simulink model "Aufgabe_9"  (Simulink 9.2)
settings: Solver=ode45  StartTime=0.0  StopTime=100.0  RelTol=1e-3  EnableMultiTasking=on
InitFcn:
  | t_save = 0.1
libraries: dspnetwork x9, simulink x2
settings Model: Creator=ST  LastModifiedBy=fleic
settings SolverCC: ZeroCrossAlgorithm=Adaptive
settings DataIOCC: SignalLoggingSaveFormat=Dataset
settings DebuggingCC: SolverPrmCheckMsg=warning  FcnCallInpInsideContextMsg=error
settings GRTTargetCC: CombineOutputUpdateFcns=on  GRTInterface=off
settings ConfigComp: CovSFcnEnable=off

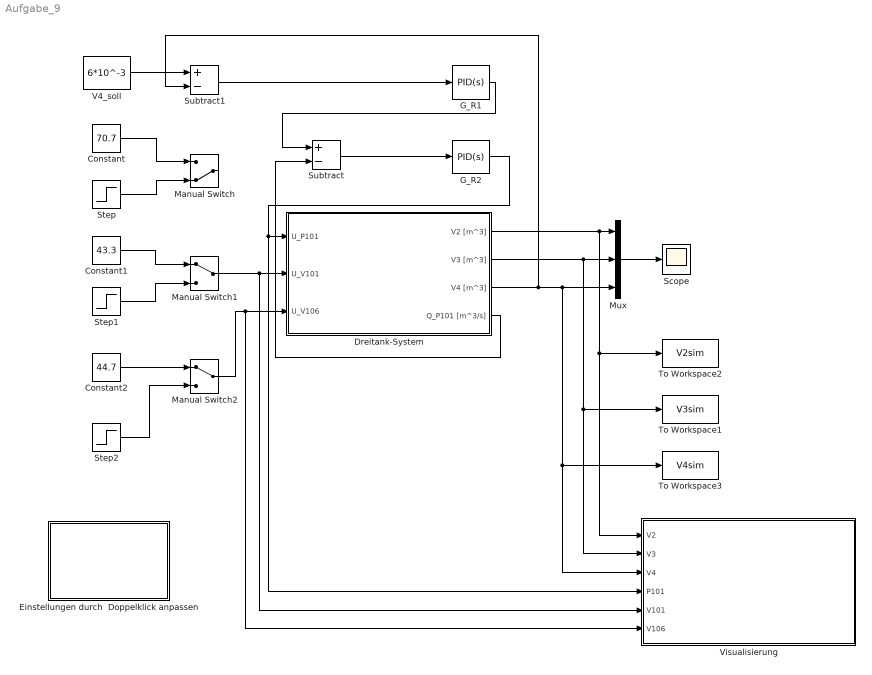
== system Aufgabe_9 ==
  Constant : Constant  Value=70.7
  Constant1 : Constant  Value=43.3
  Constant2 : Constant  Value=44.7
  Dreitank-System : Subsystem  mask{B101_Volumen=80*10^-3, B102_Initial_Volumen=8*10^-3, B103_Initial_Volumen=6*10^-3, B104_Initial_Volumen=5*10^-3, Querschnitt_Rohr_B102_B103=600*10^-6, Querschnitt_Rohr_B103_B104=600*10^-6, Flaeche_Behaelter=0.029}
      mask prompts: B101_Volumen "Volumen im Behälter B101 in m^3"; B102_Initial_Volumen "Initialvolumen im Behälter B102 in m^3"; B103_Initial_Volumen "Initialvolumen im Behälter B103 in m^3"; B104_Initial_Volumen "Initialvolumen im Behälter B104 in m^3"; Querschnitt_Rohr_B102_B103 "Rohrquerschnitt zwischen Behälter B102 und B103 in m^2"; Querschnitt_Rohr_B103_B104 "Rohrquerschnitt zwischen Behälter B103 und B104 in m^2"; Flaeche_Behaelter "Fläche der Behälter in m^2"
  Einstellungen durch  Doppelklick anpassen : MATLAB Function  InitFcn=tic  TreatAsAtomicUnit=on  mask{Auswahl=Bearbeiten}
      mask init:
      | maskStr = get_param(gcb,'Auswahl');
      | 
      | if strcmp(maskStr(1),'I')
      |      assignin('base','Testen',0)
      | else if strcmp(maskStr(1),'M')
      |         assignin('base','Testen',1)
      |     else
      |         assignin('base','Testen',2)
      |     end
      | end
  G_R1 : simulink/Continuous/PID Controller  Controller=PID  Form=Parallel  TimeDomain=Continuous-time  SampleTime=-1  IntegratorMethod=Forward Euler  FilterMethod=Forward Euler  ControllerParametersSource=internal  P=60  I=1  D=0  UseFilter=on  N=100  TunerSelectOption=Transfer Function Based (PID Tuner App)  InitialConditionSource=internal  InitialConditionForIntegrator=0  InitialConditionForFilter=0  DifferentiatorICPrevScaledInput=0  ExternalReset=none  TrackingMode=off  Kt=1  LimitOutput=off  UpperSaturationLimit=inf  LowerSaturationLimit=-inf  LinearizeAsGain=on  AntiWindupMode=none  Kb=1  POutMin=[]  POutMax=[]  IOutMin=[]  IOutMax=[]  DOutMin=[]  DOutMax=[]  NOutMin=[]  NOutMax=[]  SumOutMin=[]  SumOutMax=[]  SaturationOutMin=[]  SaturationOutMax=[]  PParamMin=[]  PParamMax=[]  IParamMin=[]  IParamMax=[]  DParamMin=[]  DParamMax=[]  NParamMin=[]  NParamMax=[]  KbParamMin=[]  KbParamMax=[]  KtParamMin=[]  KtParamMax=[]  KbOutMin=[]  KbOutMax=[]  KtOutMin=[]  KtOutMax=[]  IntegratorOutMin=[]  IntegratorOutMax=[]  FilterOutMin=[]  FilterOutMax=[]  SumI1OutMin=[]  SumI1OutMax=[]  SumI2OutMin=[]  SumI2OutMax=[]  SumI3OutMin=[]  SumI3OutMax=[]  SumI4OutMin=[]  SumI4OutMax=[]  SumDOutMin=[]  SumDOutMax=[]  DifferentiatorOutMin=[]  DifferentiatorOutMax=[]  FilterDiffOutCoefMin=[]  FilterDiffOutCoefMax=[]  ReciprocalOutMin=[]  ReciprocalOutMax=[]  SumDenOutMin=[]  SumDenOutMax=[]  SumNumOutMin=[]  SumNumOutMax=[]  DivideOutMin=[]  DivideOutMax=[]  IntegratorContinuousStateAttributes=''  IntegratorStateMustResolveToSignalObject=off  IntegratorRTWStateStorageClass=Auto  FilterContinuousStateAttributes=''  FilterStateMustResolveToSignalObject=off  FilterRTWStateStorageClass=Auto  ParallelPVariant=InternalParameters  IdealPVariant=Disabled  IVariant=InternalParameters  DVariant=InternalParameters  IntegratorVariant=Continuous  SatVariant=Disabled  AWVariant=Passthrough  PCopyVariant=Disabled  TRVariant=Disabled  FdbkBlocksVariant=Forward  IdealPFdbkVariant=Disabled  SatFdbkVariant=Disabled  DerivativeFilterVariant=ContFilter  NVariant=InternalParameters  NCopyVariant=Disabled  FilterICVariant=InternalICsFilter  IntegratorICVariant=InternalICs  ExternalResetVariant=Disabled  TRSumVariant=Passthrough  SumFdbkVariant=Disabled  SumVariant=Sum_PID
  "G_R2 " : simulink/Continuous/PID Controller  Controller=PID  Form=Parallel  TimeDomain=Continuous-time  SampleTime=-1  IntegratorMethod=Forward Euler  FilterMethod=Forward Euler  ControllerParametersSource=internal  P=469*50  I=469  D=0  UseFilter=on  N=100  TunerSelectOption=Transfer Function Based (PID Tuner App)  InitialConditionSource=internal  InitialConditionForIntegrator=0  InitialConditionForFilter=0  DifferentiatorICPrevScaledInput=0  ExternalReset=none  TrackingMode=off  Kt=1  LimitOutput=off  UpperSaturationLimit=inf  LowerSaturationLimit=-inf  LinearizeAsGain=on  AntiWindupMode=none  Kb=1  POutMin=[]  POutMax=[]  IOutMin=[]  IOutMax=[]  DOutMin=[]  DOutMax=[]  NOutMin=[]  NOutMax=[]  SumOutMin=[]  SumOutMax=[]  SaturationOutMin=[]  SaturationOutMax=[]  PParamMin=[]  PParamMax=[]  IParamMin=[]  IParamMax=[]  DParamMin=[]  DParamMax=[]  NParamMin=[]  NParamMax=[]  KbParamMin=[]  KbParamMax=[]  KtParamMin=[]  KtParamMax=[]  KbOutMin=[]  KbOutMax=[]  KtOutMin=[]  KtOutMax=[]  IntegratorOutMin=[]  IntegratorOutMax=[]  FilterOutMin=[]  FilterOutMax=[]  SumI1OutMin=[]  SumI1OutMax=[]  SumI2OutMin=[]  SumI2OutMax=[]  SumI3OutMin=[]  SumI3OutMax=[]  SumI4OutMin=[]  SumI4OutMax=[]  SumDOutMin=[]  SumDOutMax=[]  DifferentiatorOutMin=[]  DifferentiatorOutMax=[]  FilterDiffOutCoefMin=[]  FilterDiffOutCoefMax=[]  ReciprocalOutMin=[]  ReciprocalOutMax=[]  SumDenOutMin=[]  SumDenOutMax=[]  SumNumOutMin=[]  SumNumOutMax=[]  DivideOutMin=[]  DivideOutMax=[]  IntegratorContinuousStateAttributes=''  IntegratorStateMustResolveToSignalObject=off  IntegratorRTWStateStorageClass=Auto  FilterContinuousStateAttributes=''  FilterStateMustResolveToSignalObject=off  FilterRTWStateStorageClass=Auto  ParallelPVariant=InternalParameters  IdealPVariant=Disabled  IVariant=InternalParameters  DVariant=InternalParameters  IntegratorVariant=Continuous  SatVariant=Disabled  AWVariant=Passthrough  PCopyVariant=Disabled  TRVariant=Disabled  FdbkBlocksVariant=Forward  IdealPFdbkVariant=Disabled  SatFdbkVariant=Disabled  DerivativeFilterVariant=ContFilter  NVariant=InternalParameters  NCopyVariant=Disabled  FilterICVariant=InternalICsFilter  IntegratorICVariant=InternalICs  ExternalResetVariant=Disabled  TRSumVariant=Passthrough  SumFdbkVariant=Disabled  SumVariant=Sum_PID
  Manual Switch : ManualSwitch  CurrentSetting=0
  Manual Switch1 : ManualSwitch
  Manual Switch2 : ManualSwitch
  Mux : Mux  Inputs=3
  Scope : Scope
  Step : Step  Before=70.7  After=80.7  SampleTime=0
  Step1 : Step  Before=43.3  After=53.3  SampleTime=0
  Step2 : Step  Before=44.7  After=54.7  SampleTime=0
  Subtract : Sum  Inputs=+-
  Subtract1 : Sum  Inputs=+-
  To Workspace1 : ToWorkspace  VariableName=V3sim  SampleTime=t_save
  To Workspace2 : ToWorkspace  VariableName=V2sim  SampleTime=t_save
  To Workspace3 : ToWorkspace  VariableName=V4sim  SampleTime=t_save
  "V4_soll " : Constant  Value=6*10^-3
  Visualisierung : Subsystem
      settings: OpenFcn=|
      | !Dreitank_Visualisierung_64bit\Dreitank.blend.exe
      | !Dreitank_Visualisierung_32bit\Dreitank.blend.exe
  wires:
  Dreitank-System/1(V2 [m^3]) -> Visualisierung/1(V2), To Workspace2/1, Mux/1
  Dreitank-System/2(V3 [m^3]) -> Visualisierung/2(V3), To Workspace1/1, Mux/2
  Dreitank-System/3(V4 [m^3]) -> Subtract1/2, Visualisierung/3(V4), To Workspace3/1, Mux/3
  Mux/1 -> Scope/1
  Constant/1 -> Manual Switch/1
  Step/1 -> Manual Switch/2
  Manual Switch1/1 -> Dreitank-System/2("U_V101 "), Visualisierung/5(V101)
  Constant1/1 -> Manual Switch1/1
  Step1/1 -> Manual Switch1/2
  Constant2/1 -> Manual Switch2/1
  Step2/1 -> Manual Switch2/2
  Manual Switch2/1 -> Visualisierung/6(V106), Dreitank-System/3(U_V106)
  Dreitank-System/4(Q_P101 [m^3/s]) -> Subtract/2
  Subtract/1 -> "G_R2 "/1
  "G_R2 "/1 -> Visualisierung/4(P101), Dreitank-System/1(U_P101)
  "V4_soll "/1 -> Subtract1/1
  Subtract1/1 -> G_R1/1
  G_R1/1 -> Subtract/1

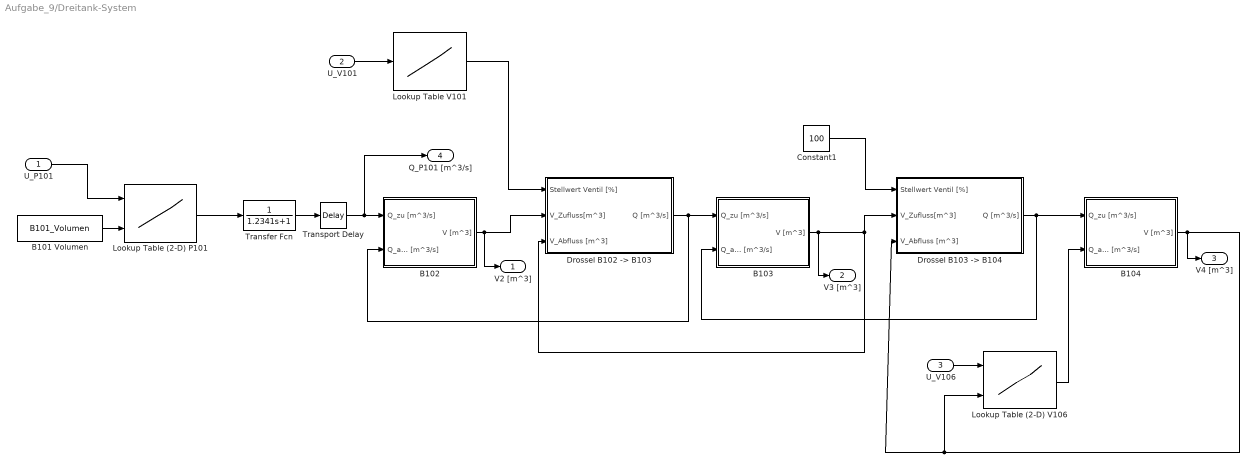
== system Aufgabe_9/Dreitank-System ==
  U_P101 : Inport
  "U_V101 " : Inport  Port=2
  U_V106 : Inport  Port=3
  B101 Volumen : Constant  Value=B101_Volumen  OutDataTypeStr=double
  B102 : Subsystem  mask{Initial_Volumen=B102_Initial_Volumen}
      mask prompts: Initial_Volumen "Initialvolumen"
  B103 : Subsystem  mask{Initial_Volumen=B103_Initial_Volumen}
      mask prompts: Initial_Volumen "Initialvolumen"
  B104 : Subsystem  mask{Initial_Volumen=B104_Initial_Volumen}
      mask prompts: Initial_Volumen "Initialvolumen"
  Constant1 : Constant  Value=100
  "Drossel B102 -> B103" : Subsystem  mask{Querschnitt_Rohr=Querschnitt_Rohr_B102_B103, Flaeche_Behaelter=Flaeche_Behaelter}
      mask prompts: Querschnitt_Rohr "Querschnitt des Rohrs in m^2"; Flaeche_Behaelter "Flaeche_Behaelter in m^2"
  "Drossel B103 -> B104" : Subsystem  mask{Querschnitt_Rohr=Querschnitt_Rohr_B102_B103, Flaeche_Behaelter=Flaeche_Behaelter}
      mask prompts: Querschnitt_Rohr "Querschnitt des Rohrs in m^2"; Flaeche_Behaelter "Flaeche_Behaelter in m^2"
  Lookup Table (2-D) P101 : Lookup2D  RowIndex=[50,55,60,65,70,75,80,85,90,95,100]  ColumnIndex=[40,130]*10^-3  Table=reshape([0,0.0606,0.2450,0.3378,0.4184,0.5002,0.5801,0.6551,0.7138,0.7746,0.8206,0,0.2799,0.3497,0.4278,0.5053,0.5810,0.6481,0.7168,0.7695,0.8350,0.8786]*10^-3,11,2)  LookUpMeth=Interpolation-Use End Values
  Lookup Table (2-D) V106 : Lookup2D  RowIndex=[15,20,25,30,35,40,45,50,55,60,65,70,75,80,85]  ColumnIndex=[2,2.8,10]*10^-3  Table=reshape([0,0,0,0,0,0,0,0,0,0,0,0,0,0,0,0,0.032,0.097,0.179,0.262,0.361,0.475,0.604,0.902,1.089,1.318,1.536,1.685,1.853,2.029,0,0.032,0.097,0.179,0.262,0.361,0.475,0.604,0.902,1.089,1.318,1.536,1.685,1.853,2.029]*10^-3,15,3)  LookUpMeth=Interpolation-Use End Values
  Lookup Table V101 : Lookup  InputValues=[0,20,25,30,35,40,45,50,55,60,65,70,75,80,85,90,100]  Table=[100,96,90,88,84,76,68,60,49,41,34,27,22,19,16,12,0]  LookUpMeth=Interpolation-Use End Values
  Transfer Fcn : TransferFcn  Denominator=[1.2341 1]
  Transport Delay : TransportDelay  DelayTime=1.1
  V2 [m^3] : Outport
  V3 [m^3] : Outport  Port=2
  V4 [m^3] : Outport  Port=3
  Q_P101 [m^3/s] : Outport  Port=4
  wires:
  "Drossel B103 -> B104"/1(Q [m^3/s]) -> B104/1(Q_zu [m^3/s]), B103/2(Q_ab [m^3/s])
  "Drossel B102 -> B103"/1(Q [m^3/s]) -> B102/2(Q_ab [m^3/s]), B103/1(Q_zu [m^3/s])
  B101 Volumen/1 -> Lookup Table (2-D) P101/2
  B103/1(V [m^3]) -> "Drossel B103 -> B104"/2(V_Zufluss[m^3]), "Drossel B102 -> B103"/3(V_Abfluss [m^3]), V3 [m^3]/1
  U_P101/1 -> Lookup Table (2-D) P101/1
  U_V106/1 -> Lookup Table (2-D) V106/1
  Lookup Table V101/1 -> "Drossel B102 -> B103"/1(Stellwert Ventil [%])
  Lookup Table (2-D) V106/1 -> B104/2(Q_ab [m^3/s])
  B102/1(V [m^3]) -> V2 [m^3]/1, "Drossel B102 -> B103"/2(V_Zufluss[m^3])
  "U_V101 "/1 -> Lookup Table V101/1
  B104/1(V [m^3]) -> Lookup Table (2-D) V106/2, "Drossel B103 -> B104"/3(V_Abfluss [m^3]), V4 [m^3]/1
  Constant1/1 -> "Drossel B103 -> B104"/1(Stellwert Ventil [%])
  Transfer Fcn/1 -> Transport Delay/1
  Lookup Table (2-D) P101/1 -> Transfer Fcn/1
  Transport Delay/1 -> Q_P101 [m^3/s]/1, B102/1(Q_zu [m^3/s])

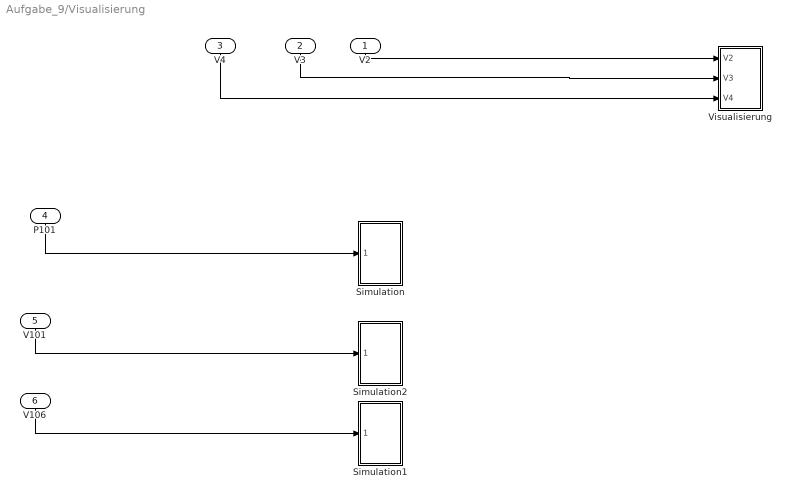
== system Aufgabe_9/Visualisierung ==
  V2 : Inport
  V3 : Inport  Port=2
  V4 : Inport  Port=3
  P101 : Inport  Port=4
  V101 : Inport  Port=5
  V106 : Inport  Port=6
  Simulation : Subsystem
  Simulation1 : Subsystem
  Simulation2 : Subsystem
  "Visualisierung " : Subsystem
      settings: OpenFcn=Visualisierung/Dreitank.exe
  wires:
  V106/1 -> Simulation1/1(ValveOne Value)
  V101/1 -> Simulation2/1(ValveTwo Value)
  V2/1 -> "Visualisierung "/1(V2)
  V4/1 -> "Visualisierung "/3("V4 ")
  P101/1 -> Simulation/1(PumpValue)
  V3/1 -> "Visualisierung "/2(V3)

== system Aufgabe_9/Dreitank-System/B102 ==
  Q_zu [m^3/s] : Inport
  Q_ab [m^3/s] : Inport  Port=2
  Integrator1 : Integrator  InitialCondition=Initial_Volumen  LimitOutput=on  UpperSaturationLimit=10*10^-3  LowerSaturationLimit=0  ContinuousStateAttributes='Volumen_B102'
  Sum : Sum  Inputs=|+-
  V [m^3] : Outport
  wires:
  Q_ab [m^3/s]/1 -> Sum/2
  Q_zu [m^3/s]/1 -> Sum/1
  Integrator1/1 -> V [m^3]/1
  Sum/1 -> Integrator1/1

== system Aufgabe_9/Dreitank-System/B103 ==
  Q_zu [m^3/s] : Inport
  Q_ab [m^3/s] : Inport  Port=2
  Integrator1 : Integrator  InitialCondition=Initial_Volumen  LimitOutput=on  UpperSaturationLimit=10*10^-3  LowerSaturationLimit=0  ContinuousStateAttributes='Volumen_B102'
  Sum : Sum  Inputs=|+-
  V [m^3] : Outport
  wires:
  Q_ab [m^3/s]/1 -> Sum/2
  Q_zu [m^3/s]/1 -> Sum/1
  Integrator1/1 -> V [m^3]/1
  Sum/1 -> Integrator1/1

== system Aufgabe_9/Dreitank-System/B104 ==
  Q_zu [m^3/s] : Inport
  Q_ab [m^3/s] : Inport  Port=2
  Integrator1 : Integrator  InitialCondition=Initial_Volumen  LimitOutput=on  UpperSaturationLimit=10*10^-3  LowerSaturationLimit=0  ContinuousStateAttributes='Volumen_B102'
  Sum : Sum  Inputs=|+-
  V [m^3] : Outport
  wires:
  Sum/1 -> Integrator1/1
  Integrator1/1 -> V [m^3]/1
  Q_zu [m^3/s]/1 -> Sum/1
  Q_ab [m^3/s]/1 -> Sum/2

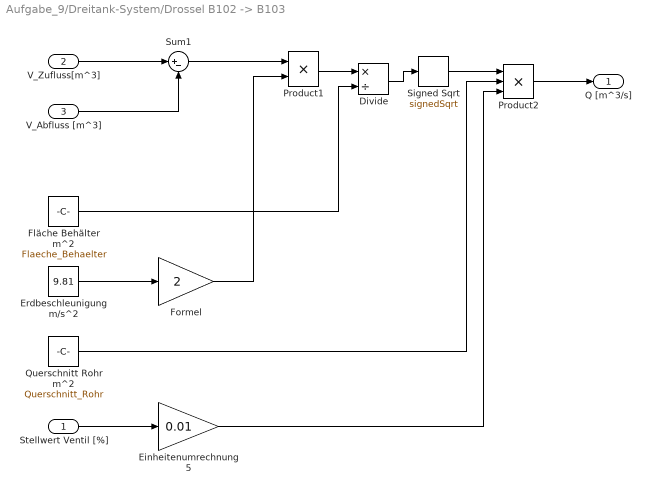
== system Aufgabe_9/Dreitank-System/Drossel B102 -> B103 ==
  Stellwert Ventil [%] : Inport
  V_Zufluss[m^3] : Inport  Port=2
  V_Abfluss [m^3] : Inport  Port=3
  Divide : Product  Inputs=*/
  Einheitenumrechnung 5 : Gain  Gain=0.01
  Erdbeschleunigung m/s^2 : Constant  Value=9.81  OutDataTypeStr=double
  Fläche Behälter m^2 : Constant  Value=Flaeche_Behaelter  OutDataTypeStr=double
  Formel : Gain  Gain=2
  Product1 : Product  RndMeth=Zero
  Product2 : Product  Inputs=3  RndMeth=Zero
  Querschnitt Rohr m^2 : Constant  Value=Querschnitt_Rohr  OutDataTypeStr=double
  Signed Sqrt : Sqrt  Operator=signedSqrt  SaturateOnIntegerOverflow=on
  Sum1 : Sum  Inputs=|+-
  Q [m^3/s] : Outport
  wires:
  Fläche Behälter m^2/1 -> Divide/2
  Divide/1 -> Signed Sqrt/1
  Product1/1 -> Divide/1
  Formel/1 -> Product1/2
  Sum1/1 -> Product1/1
  V_Abfluss [m^3]/1 -> Sum1/2
  V_Zufluss[m^3]/1 -> Sum1/1
  Product2/1 -> Q [m^3/s]/1
  Einheitenumrechnung 5/1 -> Product2/3
  Stellwert Ventil [%]/1 -> Einheitenumrechnung 5/1
  Querschnitt Rohr m^2/1 -> Product2/2
  Signed Sqrt/1 -> Product2/1
  Erdbeschleunigung m/s^2/1 -> Formel/1

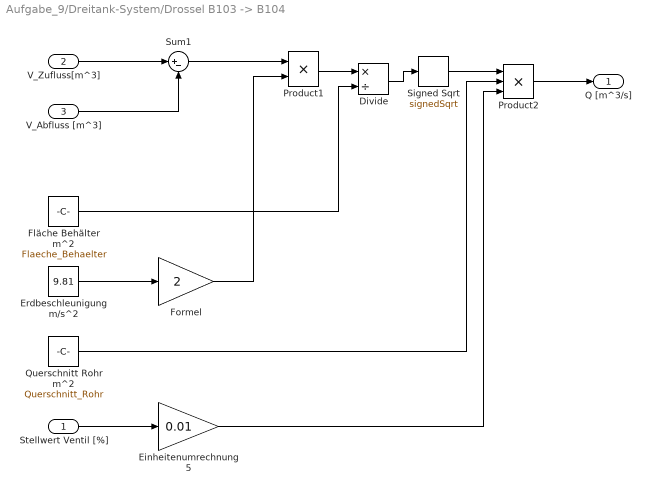
== system Aufgabe_9/Dreitank-System/Drossel B103 -> B104 ==
  Stellwert Ventil [%] : Inport
  V_Zufluss[m^3] : Inport  Port=2
  V_Abfluss [m^3] : Inport  Port=3
  Divide : Product  Inputs=*/
  Einheitenumrechnung 5 : Gain  Gain=0.01
  Erdbeschleunigung m/s^2 : Constant  Value=9.81  OutDataTypeStr=double
  Fläche Behälter m^2 : Constant  Value=Flaeche_Behaelter  OutDataTypeStr=double
  Formel : Gain  Gain=2
  Product1 : Product  RndMeth=Zero
  Product2 : Product  Inputs=3  RndMeth=Zero
  Querschnitt Rohr m^2 : Constant  Value=Querschnitt_Rohr  OutDataTypeStr=double
  Signed Sqrt : Sqrt  Operator=signedSqrt  SaturateOnIntegerOverflow=on
  Sum1 : Sum  Inputs=|+-
  Q [m^3/s] : Outport
  wires:
  Erdbeschleunigung m/s^2/1 -> Formel/1
  Signed Sqrt/1 -> Product2/1
  Querschnitt Rohr m^2/1 -> Product2/2
  Stellwert Ventil [%]/1 -> Einheitenumrechnung 5/1
  Einheitenumrechnung 5/1 -> Product2/3
  Product2/1 -> Q [m^3/s]/1
  V_Zufluss[m^3]/1 -> Sum1/1
  V_Abfluss [m^3]/1 -> Sum1/2
  Sum1/1 -> Product1/1
  Formel/1 -> Product1/2
  Product1/1 -> Divide/1
  Divide/1 -> Signed Sqrt/1
  Fläche Behälter m^2/1 -> Divide/2

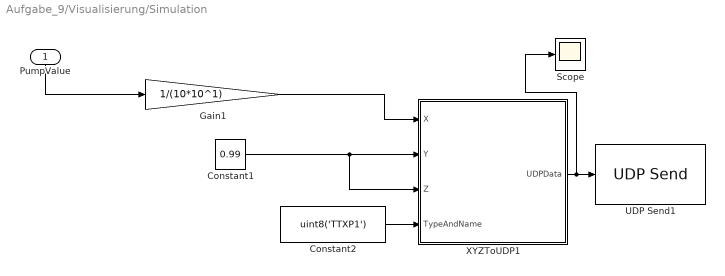
== system Aufgabe_9/Visualisierung/Simulation ==
  PumpValue : Inport
  Constant1 : Constant  Value=0.99
  Constant2 : Constant  Value=uint8('TTXP1')
  Gain1 : Gain  Gain=1/(10*10^1)
  Scope : Scope
  UDP Send1 : dspnetwork/UDP Send  remoteURL='localhost'  remotePort=9999  localURL='0.0.0.0'  localPortSource=Automatically determine  localPort=-1  sampletime=-1  blockPlatform=WINDOWS  separateLengthPort=0
      settings: SourceProductName=DSP System Toolbox  SourceProductBaseCode=DS
  XYZToUDP1 : Subsystem
  wires:
  XYZToUDP1/1(UDPData) -> Scope/1, UDP Send1/1
  Constant1/1 -> XYZToUDP1/3(Z), XYZToUDP1/2(Y)
  Constant2/1 -> XYZToUDP1/4(TypeAndName)
  PumpValue/1 -> Gain1/1
  Gain1/1 -> XYZToUDP1/1(X)

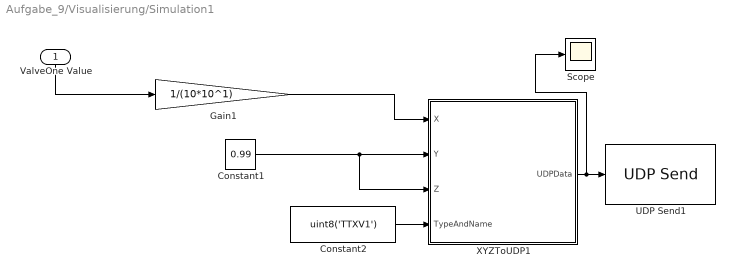
== system Aufgabe_9/Visualisierung/Simulation1 ==
  ValveOne Value : Inport
  Constant1 : Constant  Value=0.99
  Constant2 : Constant  Value=uint8('TTXV1')
  Gain1 : Gain  Gain=1/(10*10^1)
  Scope : Scope
  UDP Send1 : dspnetwork/UDP Send  remoteURL='localhost'  remotePort=9999  localURL='0.0.0.0'  localPortSource=Automatically determine  localPort=-1  sampletime=-1  blockPlatform=WINDOWS  separateLengthPort=0
      settings: SourceProductName=DSP System Toolbox  SourceProductBaseCode=DS
  XYZToUDP1 : Subsystem
  wires:
  XYZToUDP1/1(UDPData) -> Scope/1, UDP Send1/1
  Constant1/1 -> XYZToUDP1/3(Z), XYZToUDP1/2(Y)
  Constant2/1 -> XYZToUDP1/4(TypeAndName)
  ValveOne Value/1 -> Gain1/1
  Gain1/1 -> XYZToUDP1/1(X)

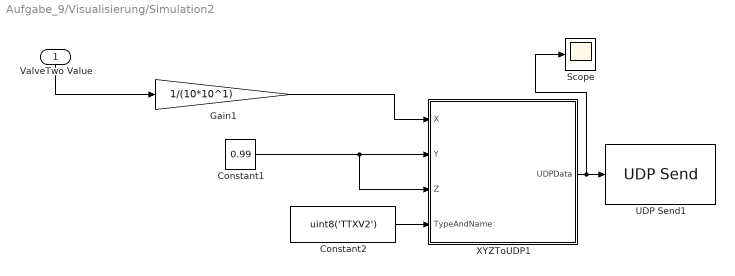
== system Aufgabe_9/Visualisierung/Simulation2 ==
  ValveTwo Value : Inport
  Constant1 : Constant  Value=0.99
  Constant2 : Constant  Value=uint8('TTXV2')
  Gain1 : Gain  Gain=1/(10*10^1)
  Scope : Scope
  UDP Send1 : dspnetwork/UDP Send  remoteURL='localhost'  remotePort=9999  localURL='0.0.0.0'  localPortSource=Automatically determine  localPort=-1  sampletime=-1  blockPlatform=WINDOWS  separateLengthPort=0
      settings: SourceProductName=DSP System Toolbox  SourceProductBaseCode=DS
  XYZToUDP1 : Subsystem
  wires:
  XYZToUDP1/1(UDPData) -> Scope/1, UDP Send1/1
  Constant1/1 -> XYZToUDP1/3(Z), XYZToUDP1/2(Y)
  Constant2/1 -> XYZToUDP1/4(TypeAndName)
  ValveTwo Value/1 -> Gain1/1
  Gain1/1 -> XYZToUDP1/1(X)

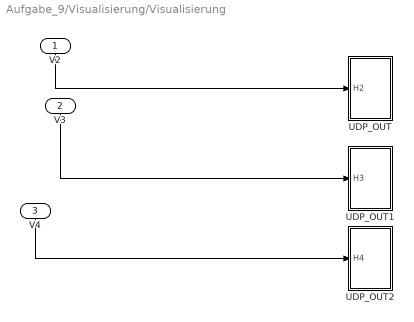
== system Aufgabe_9/Visualisierung/Visualisierung  ==
  V2 : Inport
  V3 : Inport  Port=2
  "V4 " : Inport  Port=3
  UDP_OUT : Subsystem
  UDP_OUT1 : Subsystem
  UDP_OUT2 : Subsystem
  wires:
  V2/1 -> UDP_OUT/1(H2)
  V3/1 -> UDP_OUT1/1(H3)
  "V4 "/1 -> UDP_OUT2/1(H4)

== system Aufgabe_9/Visualisierung/Simulation/XYZToUDP1 ==
  X : Inport
  Y : Inport  Port=2
  Z : Inport  Port=3
  TypeAndName : Inport  Port=4
  PrepareUDP_XYZ : MATLAB Function  TreatAsAtomicUnit=on
  UDPData : Outport
  wires:
  PrepareUDP_XYZ/1(UDPData) -> UDPData/1
  X/1 -> PrepareUDP_XYZ/1(DataX)
  TypeAndName/1 -> PrepareUDP_XYZ/4(TnName)
  Z/1 -> PrepareUDP_XYZ/3(DataZ)
  Y/1 -> PrepareUDP_XYZ/2(DataY)

== system Aufgabe_9/Visualisierung/Simulation1/XYZToUDP1 ==
  X : Inport
  Y : Inport  Port=2
  Z : Inport  Port=3
  TypeAndName : Inport  Port=4
  PrepareUDP_XYZ : MATLAB Function  TreatAsAtomicUnit=on
  UDPData : Outport
  wires:
  PrepareUDP_XYZ/1(UDPData) -> UDPData/1
  X/1 -> PrepareUDP_XYZ/1(DataX)
  TypeAndName/1 -> PrepareUDP_XYZ/4(TnName)
  Z/1 -> PrepareUDP_XYZ/3(DataZ)
  Y/1 -> PrepareUDP_XYZ/2(DataY)

== system Aufgabe_9/Visualisierung/Simulation2/XYZToUDP1 ==
  X : Inport
  Y : Inport  Port=2
  Z : Inport  Port=3
  TypeAndName : Inport  Port=4
  PrepareUDP_XYZ : MATLAB Function  TreatAsAtomicUnit=on
  UDPData : Outport
  wires:
  PrepareUDP_XYZ/1(UDPData) -> UDPData/1
  X/1 -> PrepareUDP_XYZ/1(DataX)
  TypeAndName/1 -> PrepareUDP_XYZ/4(TnName)
  Z/1 -> PrepareUDP_XYZ/3(DataZ)
  Y/1 -> PrepareUDP_XYZ/2(DataY)

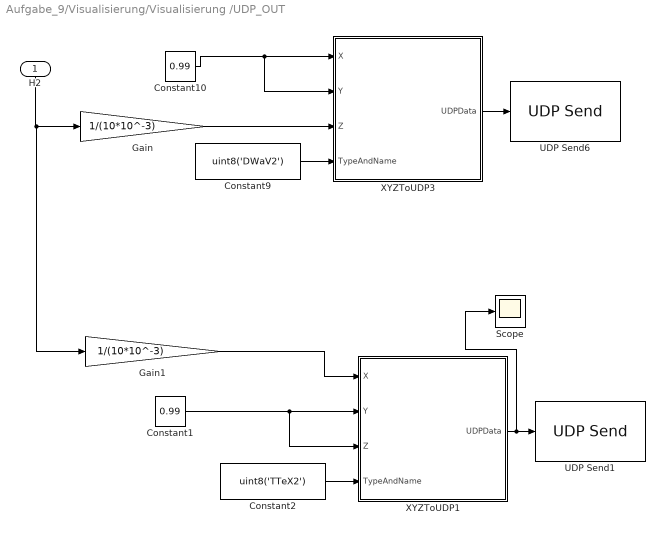
== system Aufgabe_9/Visualisierung/Visualisierung /UDP_OUT ==
  H2 : Inport
  Constant1 : Constant  Value=0.99
  Constant10 : Constant  Value=0.99
  Constant2 : Constant  Value=uint8('TTeX2')
  Constant9 : Constant  Value=uint8('DWaV2')
  Gain : Gain  Gain=1/(10*10^-3)
  Gain1 : Gain  Gain=1/(10*10^-3)
  Scope : Scope
  UDP Send1 : dspnetwork/UDP Send  remoteURL='localhost'  remotePort=9999  localURL='0.0.0.0'  localPortSource=Automatically determine  localPort=-1  sampletime=-1  blockPlatform=WINDOWS  separateLengthPort=0
      settings: SourceProductName=DSP System Toolbox  SourceProductBaseCode=DS
  UDP Send6 : dspnetwork/UDP Send  remoteURL='localhost'  remotePort=9999  localURL='0.0.0.0'  localPortSource=Automatically determine  localPort=-1  sampletime=-1  blockPlatform=WINDOWS  separateLengthPort=0
      settings: SourceProductName=DSP System Toolbox  SourceProductBaseCode=DS
  XYZToUDP1 : Subsystem
  XYZToUDP3 : Subsystem
  wires:
  XYZToUDP3/1(UDPData) -> UDP Send6/1
  Constant10/1 -> XYZToUDP3/1(X), XYZToUDP3/2(Y)
  Constant9/1 -> XYZToUDP3/4(TypeAndName)
  Gain/1 -> XYZToUDP3/3(Z)
  XYZToUDP1/1(UDPData) -> Scope/1, UDP Send1/1
  Constant1/1 -> XYZToUDP1/3(Z), XYZToUDP1/2(Y)
  Constant2/1 -> XYZToUDP1/4(TypeAndName)
  H2/1 -> Gain1/1, Gain/1
  Gain1/1 -> XYZToUDP1/1(X)

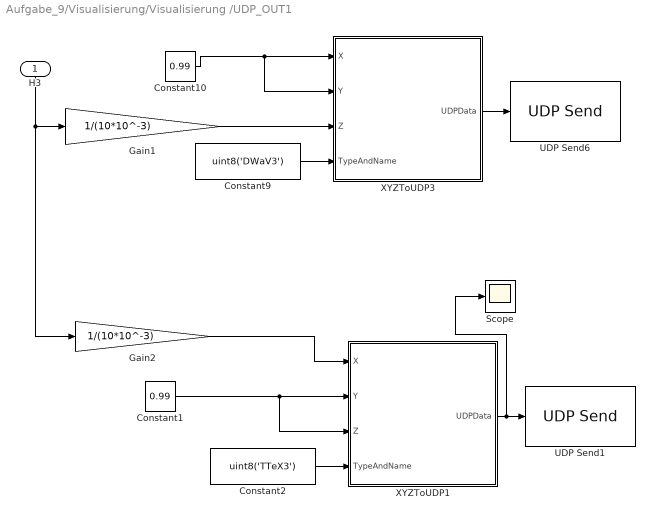
== system Aufgabe_9/Visualisierung/Visualisierung /UDP_OUT1 ==
  H3 : Inport
  Constant1 : Constant  Value=0.99
  Constant10 : Constant  Value=0.99
  Constant2 : Constant  Value=uint8('TTeX3')
  Constant9 : Constant  Value=uint8('DWaV3')
  Gain1 : Gain  Gain=1/(10*10^-3)
  Gain2 : Gain  Gain=1/(10*10^-3)
  Scope : Scope
  UDP Send1 : dspnetwork/UDP Send  remoteURL='localhost'  remotePort=9999  localURL='0.0.0.0'  localPortSource=Automatically determine  localPort=-1  sampletime=-1  blockPlatform=WINDOWS  separateLengthPort=0
      settings: SourceProductName=DSP System Toolbox  SourceProductBaseCode=DS
  UDP Send6 : dspnetwork/UDP Send  remoteURL='localhost'  remotePort=9999  localURL='0.0.0.0'  localPortSource=Automatically determine  localPort=-1  sampletime=-1  blockPlatform=WINDOWS  separateLengthPort=0
      settings: SourceProductName=DSP System Toolbox  SourceProductBaseCode=DS
  XYZToUDP1 : Subsystem
  XYZToUDP3 : Subsystem
  wires:
  XYZToUDP3/1(UDPData) -> UDP Send6/1
  Constant10/1 -> XYZToUDP3/1(X), XYZToUDP3/2(Y)
  Constant9/1 -> XYZToUDP3/4(TypeAndName)
  Gain1/1 -> XYZToUDP3/3(Z)
  XYZToUDP1/1(UDPData) -> Scope/1, UDP Send1/1
  Constant1/1 -> XYZToUDP1/3(Z), XYZToUDP1/2(Y)
  Constant2/1 -> XYZToUDP1/4(TypeAndName)
  H3/1 -> Gain2/1, Gain1/1
  Gain2/1 -> XYZToUDP1/1(X)

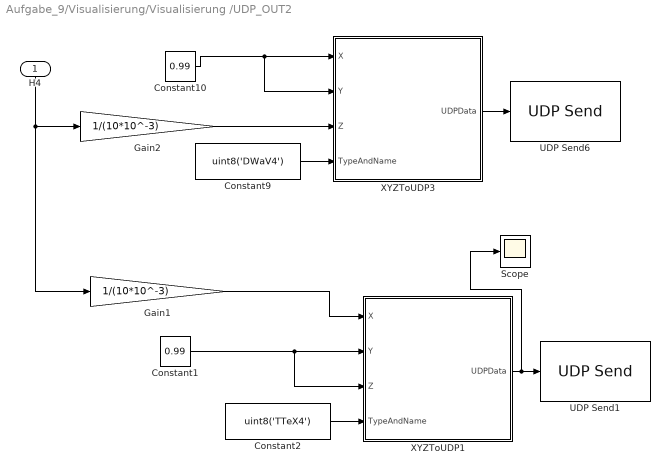
== system Aufgabe_9/Visualisierung/Visualisierung /UDP_OUT2 ==
  H4 : Inport
  Constant1 : Constant  Value=0.99
  Constant10 : Constant  Value=0.99
  Constant2 : Constant  Value=uint8('TTeX4')
  Constant9 : Constant  Value=uint8('DWaV4')
  Gain1 : Gain  Gain=1/(10*10^-3)
  Gain2 : Gain  Gain=1/(10*10^-3)
  Scope : Scope
  UDP Send1 : dspnetwork/UDP Send  remoteURL='localhost'  remotePort=9999  localURL='0.0.0.0'  localPortSource=Automatically determine  localPort=-1  sampletime=-1  blockPlatform=WINDOWS  separateLengthPort=0
      settings: SourceProductName=DSP System Toolbox  SourceProductBaseCode=DS
  UDP Send6 : dspnetwork/UDP Send  remoteURL='localhost'  remotePort=9999  localURL='0.0.0.0'  localPortSource=Automatically determine  localPort=-1  sampletime=-1  blockPlatform=WINDOWS  separateLengthPort=0
      settings: SourceProductName=DSP System Toolbox  SourceProductBaseCode=DS
  XYZToUDP1 : Subsystem
  XYZToUDP3 : Subsystem
  wires:
  XYZToUDP3/1(UDPData) -> UDP Send6/1
  Constant10/1 -> XYZToUDP3/1(X), XYZToUDP3/2(Y)
  Constant9/1 -> XYZToUDP3/4(TypeAndName)
  Gain2/1 -> XYZToUDP3/3(Z)
  XYZToUDP1/1(UDPData) -> Scope/1, UDP Send1/1
  Constant1/1 -> XYZToUDP1/3(Z), XYZToUDP1/2(Y)
  Constant2/1 -> XYZToUDP1/4(TypeAndName)
  H4/1 -> Gain1/1, Gain2/1
  Gain1/1 -> XYZToUDP1/1(X)

== system Aufgabe_9/Visualisierung/Visualisierung /UDP_OUT/XYZToUDP1 ==
  X : Inport
  Y : Inport  Port=2
  Z : Inport  Port=3
  TypeAndName : Inport  Port=4
  PrepareUDP_XYZ : MATLAB Function  TreatAsAtomicUnit=on
  UDPData : Outport
  wires:
  PrepareUDP_XYZ/1(UDPData) -> UDPData/1
  X/1 -> PrepareUDP_XYZ/1(DataX)
  TypeAndName/1 -> PrepareUDP_XYZ/4(TnName)
  Z/1 -> PrepareUDP_XYZ/3(DataZ)
  Y/1 -> PrepareUDP_XYZ/2(DataY)

== system Aufgabe_9/Visualisierung/Visualisierung /UDP_OUT/XYZToUDP3 ==
  X : Inport
  Y : Inport  Port=2
  Z : Inport  Port=3
  TypeAndName : Inport  Port=4
  PrepareUDP_XYZ : MATLAB Function  TreatAsAtomicUnit=on
  UDPData : Outport
  wires:
  PrepareUDP_XYZ/1(UDPData) -> UDPData/1
  X/1 -> PrepareUDP_XYZ/1(DataX)
  TypeAndName/1 -> PrepareUDP_XYZ/4(TnName)
  Z/1 -> PrepareUDP_XYZ/3(DataZ)
  Y/1 -> PrepareUDP_XYZ/2(DataY)

== system Aufgabe_9/Visualisierung/Visualisierung /UDP_OUT1/XYZToUDP1 ==
  X : Inport
  Y : Inport  Port=2
  Z : Inport  Port=3
  TypeAndName : Inport  Port=4
  PrepareUDP_XYZ : MATLAB Function  TreatAsAtomicUnit=on
  UDPData : Outport
  wires:
  PrepareUDP_XYZ/1(UDPData) -> UDPData/1
  X/1 -> PrepareUDP_XYZ/1(DataX)
  TypeAndName/1 -> PrepareUDP_XYZ/4(TnName)
  Z/1 -> PrepareUDP_XYZ/3(DataZ)
  Y/1 -> PrepareUDP_XYZ/2(DataY)

== system Aufgabe_9/Visualisierung/Visualisierung /UDP_OUT1/XYZToUDP3 ==
  X : Inport
  Y : Inport  Port=2
  Z : Inport  Port=3
  TypeAndName : Inport  Port=4
  PrepareUDP_XYZ : MATLAB Function  TreatAsAtomicUnit=on
  UDPData : Outport
  wires:
  PrepareUDP_XYZ/1(UDPData) -> UDPData/1
  X/1 -> PrepareUDP_XYZ/1(DataX)
  TypeAndName/1 -> PrepareUDP_XYZ/4(TnName)
  Z/1 -> PrepareUDP_XYZ/3(DataZ)
  Y/1 -> PrepareUDP_XYZ/2(DataY)

== system Aufgabe_9/Visualisierung/Visualisierung /UDP_OUT2/XYZToUDP1 ==
  X : Inport
  Y : Inport  Port=2
  Z : Inport  Port=3
  TypeAndName : Inport  Port=4
  PrepareUDP_XYZ : MATLAB Function  TreatAsAtomicUnit=on
  UDPData : Outport
  wires:
  PrepareUDP_XYZ/1(UDPData) -> UDPData/1
  X/1 -> PrepareUDP_XYZ/1(DataX)
  TypeAndName/1 -> PrepareUDP_XYZ/4(TnName)
  Z/1 -> PrepareUDP_XYZ/3(DataZ)
  Y/1 -> PrepareUDP_XYZ/2(DataY)

== system Aufgabe_9/Visualisierung/Visualisierung /UDP_OUT2/XYZToUDP3 ==
  X : Inport
  Y : Inport  Port=2
  Z : Inport  Port=3
  TypeAndName : Inport  Port=4
  PrepareUDP_XYZ : MATLAB Function  TreatAsAtomicUnit=on
  UDPData : Outport
  wires:
  PrepareUDP_XYZ/1(UDPData) -> UDPData/1
  X/1 -> PrepareUDP_XYZ/1(DataX)
  TypeAndName/1 -> PrepareUDP_XYZ/4(TnName)
  Z/1 -> PrepareUDP_XYZ/3(DataZ)
  Y/1 -> PrepareUDP_XYZ/2(DataY)

== matlab function Visualisierung/Visualisierung /UDP_OUT1/XYZToUDP3/PrepareUDP_XYZ ==
  data: DataX input double; DataY input double; DataZ input double; UDPData output uint8; TnName input double
function UDPData = XYZToBlenderUdpConversion(DataX,DataY,DataZ,TnName)
tx=typecast(single(DataX),'uint8')';
ty=typecast(single(DataY),'uint8')';
tz=typecast(single(DataZ),'uint8')';
UDPData=zeros(17,1,'uint8');
UDPData=[TnName;tx;ty;tz];

== matlab function Visualisierung/Visualisierung /UDP_OUT2/XYZToUDP3/PrepareUDP_XYZ ==
  data: DataX input double; DataY input double; DataZ input double; UDPData output uint8; TnName input double
function UDPData = XYZToBlenderUdpConversion(DataX,DataY,DataZ,TnName)
tx=typecast(single(DataX),'uint8')';
ty=typecast(single(DataY),'uint8')';
tz=typecast(single(DataZ),'uint8')';
UDPData=zeros(17,1,'uint8');
UDPData=[TnName;tx;ty;tz];

== matlab function Visualisierung/Visualisierung /UDP_OUT2/XYZToUDP1/PrepareUDP_XYZ ==
  data: DataX input double; DataY input double; DataZ input double; UDPData output uint8; TnName input double
function UDPData = XYZToBlenderUdpConversion(DataX,DataY,DataZ,TnName)
tx=typecast(single(DataX),'uint8')';
ty=typecast(single(DataY),'uint8')';
tz=typecast(single(DataZ),'uint8')';
UDPData=zeros(17,1,'uint8');
UDPData=[TnName;tx;ty;tz];

== matlab function Visualisierung/Visualisierung /UDP_OUT1/XYZToUDP1/PrepareUDP_XYZ ==
  data: DataX input double; DataY input double; DataZ input double; UDPData output uint8; TnName input double
function UDPData = XYZToBlenderUdpConversion(DataX,DataY,DataZ,TnName)
tx=typecast(single(DataX),'uint8')';
ty=typecast(single(DataY),'uint8')';
tz=typecast(single(DataZ),'uint8')';
UDPData=zeros(17,1,'uint8');
UDPData=[TnName;tx;ty;tz];

== matlab function Visualisierung/Visualisierung /UDP_OUT/XYZToUDP3/PrepareUDP_XYZ ==
  data: DataX input double; DataY input double; DataZ input double; UDPData output uint8; TnName input double
function UDPData = XYZToBlenderUdpConversion(DataX,DataY,DataZ,TnName)
tx=typecast(single(DataX),'uint8')';
ty=typecast(single(DataY),'uint8')';
tz=typecast(single(DataZ),'uint8')';
UDPData=zeros(17,1,'uint8');
UDPData=[TnName;tx;ty;tz];

== matlab function Visualisierung/Visualisierung /UDP_OUT/XYZToUDP1/PrepareUDP_XYZ ==
  data: DataX input double; DataY input double; DataZ input double; UDPData output uint8; TnName input double
function UDPData = XYZToBlenderUdpConversion(DataX,DataY,DataZ,TnName)
tx=typecast(single(DataX),'uint8')';
ty=typecast(single(DataY),'uint8')';
tz=typecast(single(DataZ),'uint8')';
UDPData=zeros(17,1,'uint8');
UDPData=[TnName;tx;ty;tz];

== matlab function Visualisierung/Simulation/XYZToUDP1/PrepareUDP_XYZ ==
  data: DataX input double; DataY input double; DataZ input double; UDPData output uint8; TnName input double
function UDPData = XYZToBlenderUdpConversion(DataX,DataY,DataZ,TnName)
tx=typecast(single(DataX),'uint8')';
ty=typecast(single(DataY),'uint8')';
tz=typecast(single(DataZ),'uint8')';
UDPData=zeros(17,1,'uint8');
UDPData=[TnName;tx;ty;tz];

== matlab function Visualisierung/Simulation1/XYZToUDP1/PrepareUDP_XYZ ==
  data: DataX input double; DataY input double; DataZ input double; UDPData output uint8; TnName input double
function UDPData = XYZToBlenderUdpConversion(DataX,DataY,DataZ,TnName)
tx=typecast(single(DataX),'uint8')';
ty=typecast(single(DataY),'uint8')';
tz=typecast(single(DataZ),'uint8')';
UDPData=zeros(17,1,'uint8');
UDPData=[TnName;tx;ty;tz];

== matlab function Visualisierung/Simulation2/XYZToUDP1/PrepareUDP_XYZ ==
  data: DataX input double; DataY input double; DataZ input double; UDPData output uint8; TnName input double
function UDPData = XYZToBlenderUdpConversion(DataX,DataY,DataZ,TnName)
tx=typecast(single(DataX),'uint8')';
ty=typecast(single(DataY),'uint8')';
tz=typecast(single(DataZ),'uint8')';
UDPData=zeros(17,1,'uint8');
UDPData=[TnName;tx;ty;tz];

== matlab function Einstellungen durch Doppelklick anpassen ==
  settings: updateMethod=DISCRETE  sampleTime=0.1
function Auswahl


coder.extrinsic('tic');
coder.extrinsic('toc');
coder.extrinsic('drawnow');
coder.extrinsic('evalin');

Testen = 0;
Testen = evalin('base','Testen');

if Testen == 0

    t = 0;
    t = toc;
    while t < 0.1
    t = toc;
    drawnow;
    end
    tic;

end
